simulink model "lineal_closeloop_X2_comp"  (Simulink 7.9)
settings: Solver=ode3  StartTime=0.0  StopTime=80  FixedStep=1  RelTol=1e-3
libraries: simulink x3
settings Model: Creator=JuanPablo  LastModifiedBy=JuanPablo

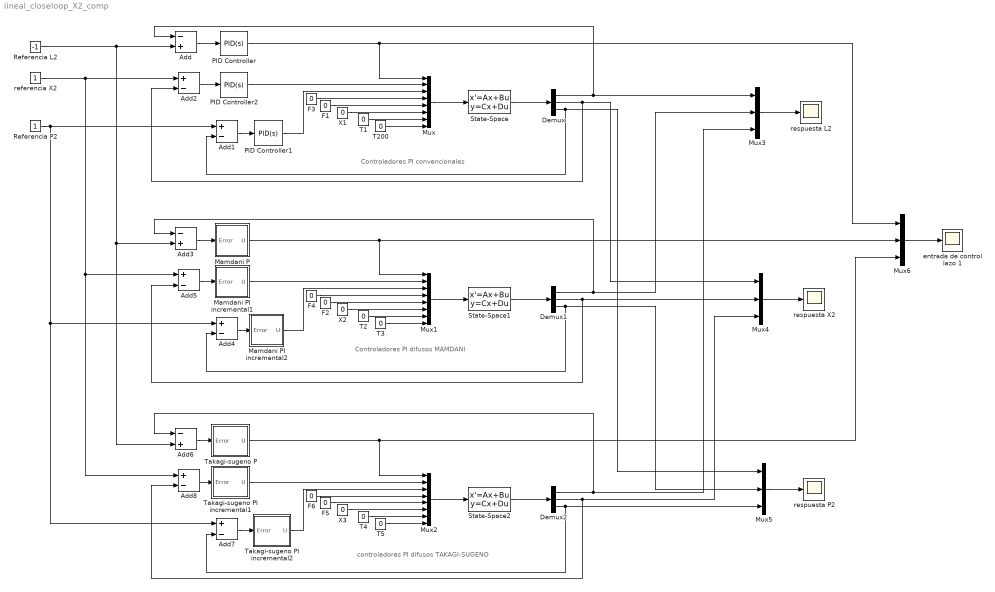
== system lineal_closeloop_X2_comp ==
  note: Controladores PI difusos MAMDANI
  note: controladores PI difusos TAKAGI-SUGENO
  note: Controladores PI convencionales
  Add : Sum  Inputs=-+
  Add{1..2,4..5,7..8} (6 alike) : Sum  Inputs=+-
  Add3 : Sum  Inputs=-+
  Add6 : Sum  Inputs=-+
  Demux : Demux  Outputs=3
  Demux1 : Demux  Outputs=3
  Demux2 : Demux  Outputs=3
  F{1..6} (6 alike) : Constant  Value=0
  Mamdani P : Subsystem  TreatAsAtomicUnit=on  mask{GE=1, GU=-7.5}
  Mamdani PI incremental1 : Subsystem  TreatAsAtomicUnit=on  mask{GE=1, GCE=2.664, GCU=1.39066}
  Mamdani PI incremental2 : Subsystem  TreatAsAtomicUnit=on  mask{GE=1, GCE=10.989, GCU=-3.87779}
  Mux : Mux  Inputs=8
  Mux1 : Mux  Inputs=8
  Mux2 : Mux  Inputs=8
  Mux{3..6} (4 alike) : Mux  Inputs=3
  PID Controller : simulink/Continuous/PID Controller  Controller=PID  TimeDomain=Continuous-time  SampleTime=1  IntegratorMethod=Forward Euler  FilterMethod=Forward Euler  Form=Parallel  P=-7.5  I=0  D=0  N=100  InitialConditionSource=internal  InitialConditionForIntegrator=0  InitialConditionForFilter=0  ExternalReset=none  LimitOutput=off  UpperSaturationLimit=inf  LowerSaturationLimit=-inf  LinearizeAsGain=off  AntiWindupMode=none  Kb=1  TrackingMode=off  Kt=1  PParamMin=[]  PParamMax=[]  IParamMin=[]  IParamMax=[]  DParamMin=[]  DParamMax=[]  NParamMin=[]  NParamMax=[]  KbParamMin=[]  KbParamMax=[]  KtParamMin=[]  KtParamMax=[]  POutMin=[]  POutMax=[]  IOutMin=[]  IOutMax=[]  DOutMin=[]  DOutMax=[]  NOutMin=[]  NOutMax=[]  KbOutMin=[]  KbOutMax=[]  KtOutMin=[]  KtOutMax=[]  IntegratorOutMin=[]  IntegratorOutMax=[]  FilterOutMin=[]  FilterOutMax=[]  SumOutMin=[]  SumOutMax=[]  SumI1OutMin=[]  SumI1OutMax=[]  SumI2OutMin=[]  SumI2OutMax=[]  SumI3OutMin=[]  SumI3OutMax=[]  SumDOutMin=[]  SumDOutMax=[]  SaturationOutMin=[]  SaturationOutMax=[]  IntegratorContinuousStateAttributes=''  IntegratorStateMustResolveToSignalObject=off  IntegratorRTWStateStorageClass=Auto  FilterContinuousStateAttributes=''  FilterStateMustResolveToSignalObject=off  FilterRTWStateStorageClass=Auto
  PID Controller1 : simulink/Continuous/PID Controller  Controller=PID  TimeDomain=Continuous-time  SampleTime=1  IntegratorMethod=Forward Euler  FilterMethod=Forward Euler  Form=Parallel  P=-42.61364  I=-42.61364/10.989  D=0  N=100  InitialConditionSource=internal  InitialConditionForIntegrator=0  InitialConditionForFilter=0  ExternalReset=none  LimitOutput=off  UpperSaturationLimit=inf  LowerSaturationLimit=-inf  LinearizeAsGain=off  AntiWindupMode=none  Kb=1  TrackingMode=off  Kt=1  PParamMin=[]  PParamMax=[]  IParamMin=[]  IParamMax=[]  DParamMin=[]  DParamMax=[]  NParamMin=[]  NParamMax=[]  KbParamMin=[]  KbParamMax=[]  KtParamMin=[]  KtParamMax=[]  POutMin=[]  POutMax=[]  IOutMin=[]  IOutMax=[]  DOutMin=[]  DOutMax=[]  NOutMin=[]  NOutMax=[]  KbOutMin=[]  KbOutMax=[]  KtOutMin=[]  KtOutMax=[]  IntegratorOutMin=[]  IntegratorOutMax=[]  FilterOutMin=[]  FilterOutMax=[]  SumOutMin=[]  SumOutMax=[]  SumI1OutMin=[]  SumI1OutMax=[]  SumI2OutMin=[]  SumI2OutMax=[]  SumI3OutMin=[]  SumI3OutMax=[]  SumDOutMin=[]  SumDOutMax=[]  SaturationOutMin=[]  SaturationOutMax=[]  IntegratorContinuousStateAttributes=''  IntegratorStateMustResolveToSignalObject=off  IntegratorRTWStateStorageClass=Auto  FilterContinuousStateAttributes=''  FilterStateMustResolveToSignalObject=off  FilterRTWStateStorageClass=Auto
  PID Controller2 : simulink/Continuous/PID Controller  Controller=PID  TimeDomain=Continuous-time  SampleTime=1  IntegratorMethod=Forward Euler  FilterMethod=Forward Euler  Form=Parallel  P=3.70472  I=3.70472/2.664  D=0  N=100  InitialConditionSource=internal  InitialConditionForIntegrator=0  InitialConditionForFilter=0  ExternalReset=none  LimitOutput=off  UpperSaturationLimit=inf  LowerSaturationLimit=-inf  LinearizeAsGain=off  AntiWindupMode=none  Kb=1  TrackingMode=off  Kt=1  PParamMin=[]  PParamMax=[]  IParamMin=[]  IParamMax=[]  DParamMin=[]  DParamMax=[]  NParamMin=[]  NParamMax=[]  KbParamMin=[]  KbParamMax=[]  KtParamMin=[]  KtParamMax=[]  POutMin=[]  POutMax=[]  IOutMin=[]  IOutMax=[]  DOutMin=[]  DOutMax=[]  NOutMin=[]  NOutMax=[]  KbOutMin=[]  KbOutMax=[]  KtOutMin=[]  KtOutMax=[]  IntegratorOutMin=[]  IntegratorOutMax=[]  FilterOutMin=[]  FilterOutMax=[]  SumOutMin=[]  SumOutMax=[]  SumI1OutMin=[]  SumI1OutMax=[]  SumI2OutMin=[]  SumI2OutMax=[]  SumI3OutMin=[]  SumI3OutMax=[]  SumDOutMin=[]  SumDOutMax=[]  SaturationOutMin=[]  SaturationOutMax=[]  IntegratorContinuousStateAttributes=''  IntegratorStateMustResolveToSignalObject=off  IntegratorRTWStateStorageClass=Auto  FilterContinuousStateAttributes=''  FilterStateMustResolveToSignalObject=off  FilterRTWStateStorageClass=Auto
  Referencia L2 : Constant  Value=-1
  Referencia P2 : Constant
  State-Space : StateSpace  A=[0 0.10455 0.37935; 0 -0.1 0; 0 -0.10340e-1 -0.54738e-1]  B=[-0.1 -0.37266 0 -0.36676 0.38605 0 -0.3636e-1 0; -0.1 0 0 0 0.1 0.1 0 0; 0 0.36914e-1 -0.75272e-2 0.36302e-1 0.32268e-2 0 0.35972e-2 0.17785e-1]  C=[1 0 0; 0 1 0; 0 0 1]  D=zeros(3,8)  ContinuousStateAttributes=['L2' 'X2' 'P2']
  State-Space1 : StateSpace  A=[0 0.10455 0.37935; 0 -0.1 0; 0 -0.10340e-1 -0.54738e-1]  B=[-0.1 -0.37266 0 -0.36676 0.38605 0 -0.3636e-1 0; -0.1 0 0 0 0.1 0.1 0 0; 0 0.36914e-1 -0.75272e-2 0.36302e-1 0.32268e-2 0 0.35972e-2 0.17785e-1]  C=[1 0 0; 0 1 0; 0 0 1]  D=zeros(3,8)  ContinuousStateAttributes=['L2' 'X2' 'P2']
  State-Space2 : StateSpace  A=[0 0.10455 0.37935; 0 -0.1 0; 0 -0.10340e-1 -0.54738e-1]  B=[-0.1 -0.37266 0 -0.36676 0.38605 0 -0.3636e-1 0; -0.1 0 0 0 0.1 0.1 0 0; 0 0.36914e-1 -0.75272e-2 0.36302e-1 0.32268e-2 0 0.35972e-2 0.17785e-1]  C=[1 0 0; 0 1 0; 0 0 1]  D=zeros(3,8)  ContinuousStateAttributes=['L2' 'X2' 'P2']
  T{1..5,200} (6 alike) : Constant  Value=0
  Takagi-sugeno P : Subsystem  TreatAsAtomicUnit=on  mask{GE=1, GU=-7.5}
  Takagi-sugeno PI incremental1 : Subsystem  TreatAsAtomicUnit=on  mask{GE=1, GCE=2.644, GCU=1.39}
  Takagi-sugeno PI incremental2 : Subsystem  TreatAsAtomicUnit=on  mask{GE=1, GCE=10.989, GCU=-3.87779}
  X1 : Constant  Value=0
  X2 : Constant  Value=0
  X3 : Constant  Value=0
  entrada de control lazo 1 : Scope
      settings: TimeRange=80  YMin=-12  YMax=8  SaveName=closeloop_u_F2
  referencia X2 : Constant
  respuesta L2 : Scope
      settings: TimeRange=80  YMin=-2.5  YMax=0  SaveName=closeloop_L2
  respuesta P2 : Scope
      settings: TimeRange=80  YMin=0  YMax=1.4  SaveName=closeloop_P2
  respuesta X2 : Scope
      settings: TimeRange=80  YMin=-1  YMax=2  SaveName=closeloop_X2
  wires:
  Mux/1 -> State-Space/1
  State-Space/1 -> Demux/1
  PID Controller2/1 -> Mux/2
  F3/1 -> Mux/4
  F1/1 -> Mux/5
  X1/1 -> Mux/6
  T1/1 -> Mux/7
  T200/1 -> Mux/8
  Demux/1 -> Add/1, Mux3/1
  Demux/2 -> Add2/2, Mux4/1
  Add/1 -> PID Controller/1
  Referencia L2/1 -> Add/2, Add3/2, Add6/2
  Referencia P2/1 -> Add1/1, Add4/1, Add7/1
  Add1/1 -> PID Controller1/1
  PID Controller1/1 -> Mux/3
  referencia X2/1 -> Add2/1, Add8/1, Add5/1
  Add2/1 -> PID Controller2/1
  PID Controller/1 -> Mux/1, Mux6/1
  Demux/3 -> Add1/2, Mux5/1
  Mux1/1 -> State-Space1/1
  State-Space1/1 -> Demux1/1
  Mamdani PI incremental1/1(U) -> Mux1/2
  F4/1 -> Mux1/4
  F2/1 -> Mux1/5
  X2/1 -> Mux1/6
  T2/1 -> Mux1/7
  T3/1 -> Mux1/8
  Demux1/1 -> Add3/1, Mux3/2
  Demux1/2 -> Add5/2, Mux4/2
  Add3/1 -> Mamdani P/1(Error)
  Add4/1 -> Mamdani PI incremental2/1(Error)
  Mamdani PI incremental2/1(U) -> Mux1/3
  Add5/1 -> Mamdani PI incremental1/1(Error)
  Mamdani P/1(U) -> Mux1/1, Mux6/2
  Demux1/3 -> Add4/2, Mux5/2
  Mux2/1 -> State-Space2/1
  State-Space2/1 -> Demux2/1
  Takagi-sugeno PI incremental1/1(U) -> Mux2/2
  F6/1 -> Mux2/4
  F5/1 -> Mux2/5
  X3/1 -> Mux2/6
  T4/1 -> Mux2/7
  T5/1 -> Mux2/8
  Demux2/1 -> Add6/1, Mux3/3
  Demux2/2 -> Add8/2, Mux4/3
  Add6/1 -> Takagi-sugeno P/1(Error)
  Add7/1 -> Takagi-sugeno PI incremental2/1(Error)
  Takagi-sugeno PI incremental2/1(U) -> Mux2/3
  Add8/1 -> Takagi-sugeno PI incremental1/1(Error)
  Takagi-sugeno P/1(U) -> Mux2/1, Mux6/3
  Demux2/3 -> Add7/2, Mux5/3
  Mux3/1 -> respuesta L2/1
  Mux4/1 -> respuesta X2/1
  Mux5/1 -> respuesta P2/1
  Mux6/1 -> entrada de control lazo 1/1

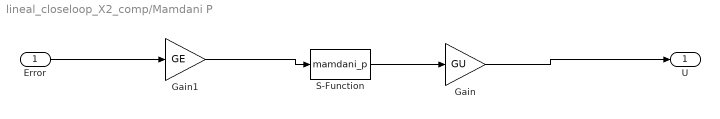
== system lineal_closeloop_X2_comp/Mamdani P ==
  Error : Inport
  Gain : Gain  Gain=GU
  Gain1 : Gain  Gain=GE
  S-Function : S-Function  FunctionName=mamdani_p  EnableBusSupport=off
  U : Outport
  wires:
  Error/1 -> Gain1/1
  Gain/1 -> U/1
  S-Function/1 -> Gain/1
  Gain1/1 -> S-Function/1

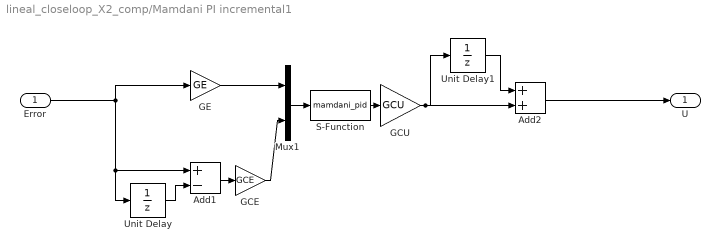
== system lineal_closeloop_X2_comp/Mamdani PI incremental1 ==
  Error : Inport
  Add1 : Sum  Inputs=+-
  Add2 : Sum
  GCE : Gain  Gain=GCE
  GCU : Gain  Gain=GCU
  GE : Gain  Gain=GE
  Mux1 : Mux  Inputs=2
  S-Function : S-Function  FunctionName=mamdani_pid  EnableBusSupport=off
  Unit Delay : UnitDelay
  Unit Delay1 : UnitDelay
  U : Outport
  wires:
  Add2/1 -> U/1
  Error/1 -> Add1/1, Unit Delay/1, GE/1
  Mux1/1 -> S-Function/1
  Unit Delay/1 -> Add1/2
  GCU/1 -> Add2/2, Unit Delay1/1
  S-Function/1 -> GCU/1
  Add1/1 -> GCE/1
  GCE/1 -> Mux1/2
  Unit Delay1/1 -> Add2/1
  GE/1 -> Mux1/1

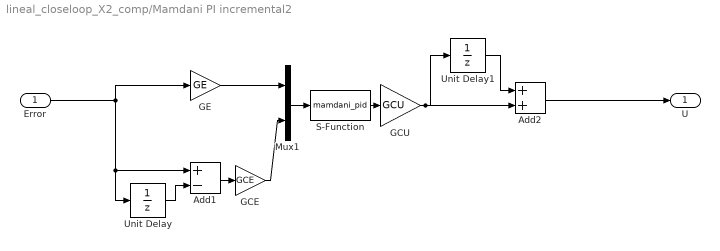
== system lineal_closeloop_X2_comp/Mamdani PI incremental2 ==
  Error : Inport
  Add1 : Sum  Inputs=+-
  Add2 : Sum
  GCE : Gain  Gain=GCE
  GCU : Gain  Gain=GCU
  GE : Gain  Gain=GE
  Mux1 : Mux  Inputs=2
  S-Function : S-Function  FunctionName=mamdani_pid  EnableBusSupport=off
  Unit Delay : UnitDelay
  Unit Delay1 : UnitDelay
  U : Outport
  wires:
  Add2/1 -> U/1
  Error/1 -> Add1/1, Unit Delay/1, GE/1
  Mux1/1 -> S-Function/1
  Unit Delay/1 -> Add1/2
  GCU/1 -> Add2/2, Unit Delay1/1
  S-Function/1 -> GCU/1
  Add1/1 -> GCE/1
  GCE/1 -> Mux1/2
  Unit Delay1/1 -> Add2/1
  GE/1 -> Mux1/1

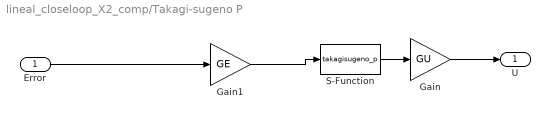
== system lineal_closeloop_X2_comp/Takagi-sugeno P ==
  Error : Inport
  Gain : Gain  Gain=GU
  Gain1 : Gain  Gain=GE
  S-Function : S-Function  FunctionName=takagisugeno_p  EnableBusSupport=off
  U : Outport
  wires:
  Error/1 -> Gain1/1
  Gain/1 -> U/1
  S-Function/1 -> Gain/1
  Gain1/1 -> S-Function/1

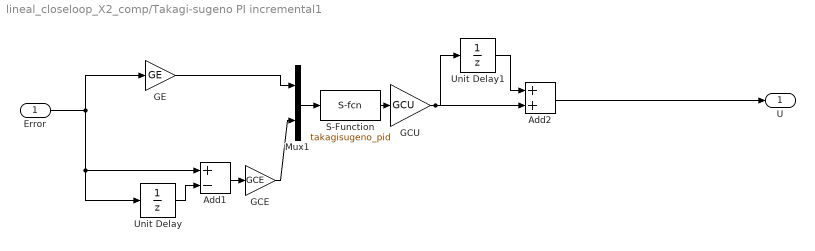
== system lineal_closeloop_X2_comp/Takagi-sugeno PI incremental1 ==
  Error : Inport
  Add1 : Sum  Inputs=+-
  Add2 : Sum
  GCE : Gain  Gain=GCE
  GCU : Gain  Gain=GCU
  GE : Gain  Gain=GE
  Mux1 : Mux  Inputs=2
  S-Function : S-Function  FunctionName=takagisugeno_pid  EnableBusSupport=off
  Unit Delay : UnitDelay
  Unit Delay1 : UnitDelay
  U : Outport
  wires:
  Add2/1 -> U/1
  Mux1/1 -> S-Function/1
  Unit Delay/1 -> Add1/2
  GCU/1 -> Add2/2, Unit Delay1/1
  S-Function/1 -> GCU/1
  Add1/1 -> GCE/1
  GCE/1 -> Mux1/2
  Unit Delay1/1 -> Add2/1
  Error/1 -> Add1/1, Unit Delay/1, GE/1
  GE/1 -> Mux1/1

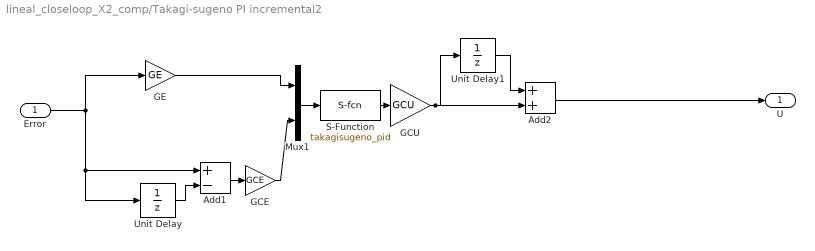
== system lineal_closeloop_X2_comp/Takagi-sugeno PI incremental2 ==
  Error : Inport
  Add1 : Sum  Inputs=+-
  Add2 : Sum
  GCE : Gain  Gain=GCE
  GCU : Gain  Gain=GCU
  GE : Gain  Gain=GE
  Mux1 : Mux  Inputs=2
  S-Function : S-Function  FunctionName=takagisugeno_pid  EnableBusSupport=off
  Unit Delay : UnitDelay
  Unit Delay1 : UnitDelay
  U : Outport
  wires:
  Add2/1 -> U/1
  Mux1/1 -> S-Function/1
  Unit Delay/1 -> Add1/2
  GCU/1 -> Add2/2, Unit Delay1/1
  S-Function/1 -> GCU/1
  Add1/1 -> GCE/1
  GCE/1 -> Mux1/2
  Unit Delay1/1 -> Add2/1
  Error/1 -> Add1/1, Unit Delay/1, GE/1
  GE/1 -> Mux1/1
